simulink model "artedoa_integration_2"  (R2013b)
settings: Solver=ode45  StartTime=0.0  StopTime=1000000  RelTol=1e-3
undefined symbols (not defined in the file or in its folder): calan_lib, comp_addsub
libraries: xbsIndex_r4 x523, casper_library_misc x77, xps_library x1
(part 1 of 2)
settings Model: Creator=root  LastModifiedBy=root

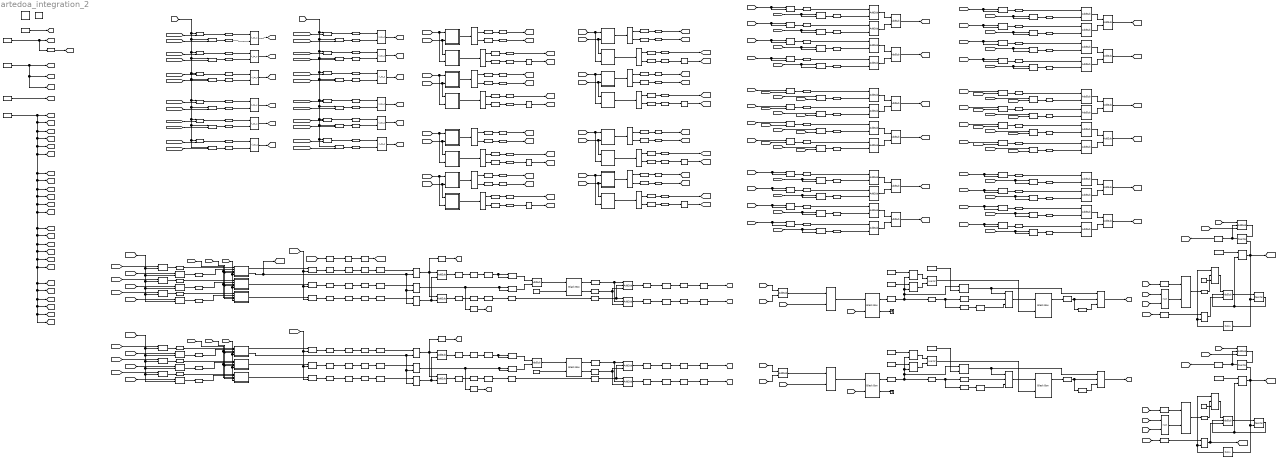
== system artedoa_integration_2 ==
  " System Generator" : xbsIndex_r4/ System Generator  Tag=genX  xilinxfamily=virtex6  part=xc6vsx475t  speed=-1  package=ff1759  synthesis_tool=XST  clock_wrapper=Clock Enables  directory=./doa2dcal/sysgen  proj_type=Project Navigator  Synth_file=XST Defaults  Impl_file=ISE Defaults  testbench=off  simulink_period=1  sysclk_period=7.1429  dcm_input_clock_period=100  incr_netlist=off  trim_vbits=Everywhere in SubSystem  dbl_ovrd=According to Block Masks  core_generation=According to Block Masks  run_coregen=off  deprecated_control=off  eval_field=0  block_type=sysgen
  AddSub : xbsIndex_r4/AddSub  mode=Addition  use_carryin=off  use_carryout=off  en=on  latency=1  precision=User Defined  arith_type="Signed  (2's comp)"  n_bits=26  bin_pt=8  quantization="Round  (unbiased: +/- Inf)"  overflow=Saturate  dbl_ovrd=off  use_behavioral_HDL=off  hw_selection=Fabric  pipelined=off  block_type=addsub
  AddSub1 : xbsIndex_r4/AddSub  mode=Addition  use_carryin=off  use_carryout=off  en=on  latency=1  precision=User Defined  arith_type=Unsigned  n_bits=10  bin_pt=0  quantization="Round  (unbiased: +/- Inf)"  overflow=Saturate  dbl_ovrd=off  use_behavioral_HDL=off  hw_selection=Fabric  pipelined=off  block_type=addsub
  AddSub{2..5,8..11,14..15,18..21,24..25,28..33,36..37} (24 alike) : xbsIndex_r4/AddSub  mode=Addition  use_carryin=off  use_carryout=off  en=off  latency=0  precision=Full  arith_type="Signed  (2's comp)"  n_bits=9  bin_pt=7  quantization="Round  (unbiased: +/- Inf)"  overflow=Saturate  dbl_ovrd=off  use_behavioral_HDL=off  hw_selection=Fabric  pipelined=off  block_type=addsub
  AddSub{6..7,12..13,16..17,22..23,26..27,34..35} (12 alike) : xbsIndex_r4/AddSub  mode=Addition  use_carryin=off  use_carryout=off  en=off  latency=0  precision=Full  arith_type="Signed  (2's comp)"  n_bits=10  bin_pt=7  quantization="Round  (unbiased: +/- Inf)"  overflow=Saturate  dbl_ovrd=off  use_behavioral_HDL=off  hw_selection=Fabric  pipelined=off  block_type=addsub
  AddSub38 : xbsIndex_r4/AddSub  mode=Addition  use_carryin=off  use_carryout=off  en=on  latency=1  precision=User Defined  arith_type="Signed  (2's comp)"  n_bits=26  bin_pt=8  quantization="Round  (unbiased: +/- Inf)"  overflow=Saturate  dbl_ovrd=off  use_behavioral_HDL=off  hw_selection=Fabric  pipelined=off  block_type=addsub
  AddSub39 : xbsIndex_r4/AddSub  mode=Addition  use_carryin=off  use_carryout=off  en=on  latency=1  precision=User Defined  arith_type=Unsigned  n_bits=10  bin_pt=0  quantization="Round  (unbiased: +/- Inf)"  overflow=Saturate  dbl_ovrd=off  use_behavioral_HDL=off  hw_selection=Fabric  pipelined=off  block_type=addsub
  Black Box : xbsIndex_r4/Black Box  init_code=arcsin_config  sim_method=ISE Simulator  verbose=off  block_type=blackbox2
  Black Box1 : xbsIndex_r4/Black Box  init_code=arcsin_config  sim_method=ISE Simulator  verbose=off  block_type=blackbox2
  Constant : xbsIndex_r4/Constant  const=1  gui_display_data_type=Boolean  arith_type=Boolean  n_bits=16  bin_pt=14  preci_type=Single  exp_width=8  frac_width=24  explicit_period=on  period=1  equ=P=C  opselect=C  inp2=PCIN>>17  opr=+  inp1=P  carry=CIN  dbl_ovrd=off  block_type=constant
  Constant1 : xbsIndex_r4/Constant  const=1  gui_display_data_type=Boolean  arith_type=Boolean  n_bits=16  bin_pt=14  preci_type=Single  exp_width=8  frac_width=24  explicit_period=off  period=1  equ=P=C  opselect=C  inp2=PCIN>>17  opr=+  inp1=P  carry=CIN  dbl_ovrd=off  block_type=constant
  Constant10 : xbsIndex_r4/Constant  const=0  gui_display_data_type=Fixed-point  arith_type=Signed (2's comp)  n_bits=16  bin_pt=12  preci_type=Single  exp_width=8  frac_width=24  explicit_period=on  period=1  equ=P=C  opselect=C  inp2=PCIN>>17  opr=+  inp1=P  carry=CIN  dbl_ovrd=off  block_type=constant
  Constant11 : xbsIndex_r4/Constant  const=16  gui_display_data_type=Fixed-point  arith_type=Unsigned  n_bits=10  bin_pt=0  preci_type=Single  exp_width=8  frac_width=24  explicit_period=on  period=1  equ=P=C  opselect=C  inp2=PCIN>>17  opr=+  inp1=P  carry=CIN  dbl_ovrd=off  block_type=constant
  Constant12 : xbsIndex_r4/Constant  const=0  gui_display_data_type=Fixed-point  arith_type=Unsigned  n_bits=1  bin_pt=0  preci_type=Single  exp_width=8  frac_width=24  explicit_period=on  period=1  equ=P=C  opselect=C  inp2=PCIN>>17  opr=+  inp1=P  carry=CIN  dbl_ovrd=off  block_type=constant
  Constant13 : xbsIndex_r4/Constant  const=1  gui_display_data_type=Fixed-point  arith_type=Unsigned  n_bits=7  bin_pt=0  preci_type=Single  exp_width=8  frac_width=24  explicit_period=on  period=1  equ=P=C  opselect=C  inp2=PCIN>>17  opr=+  inp1=P  carry=CIN  dbl_ovrd=off  block_type=constant
  Constant14 : xbsIndex_r4/Constant  const=1  gui_display_data_type=Fixed-point  arith_type=Unsigned  n_bits=9  bin_pt=4  preci_type=Single  exp_width=8  frac_width=24  explicit_period=on  period=1  equ=P=C  opselect=C  inp2=PCIN>>17  opr=+  inp1=P  carry=CIN  dbl_ovrd=off  block_type=constant
  Constant15 : xbsIndex_r4/Constant  const=1  gui_display_data_type=Fixed-point  arith_type=Unsigned  n_bits=18  bin_pt=17  preci_type=Single  exp_width=8  frac_width=24  explicit_period=on  period=1  equ=P=C  opselect=C  inp2=PCIN>>17  opr=+  inp1=P  carry=CIN  dbl_ovrd=off  block_type=constant
  Constant2 : xbsIndex_r4/Constant  const=1  gui_display_data_type=Boolean  arith_type=Boolean  n_bits=16  bin_pt=14  preci_type=Single  exp_width=8  frac_width=24  explicit_period=off  period=1  equ=P=C  opselect=C  inp2=PCIN>>17  opr=+  inp1=P  carry=CIN  dbl_ovrd=off  block_type=constant
  Constant21 : xbsIndex_r4/Constant  const=10000  gui_display_data_type=Fixed-point  arith_type=Unsigned  n_bits=20  bin_pt=0  preci_type=Single  exp_width=8  frac_width=24  explicit_period=on  period=1  equ=P=C  opselect=C  inp2=PCIN>>17  opr=+  inp1=P  carry=CIN  dbl_ovrd=off  block_type=constant
  Constant3 : xbsIndex_r4/Constant  const=1  gui_display_data_type=Fixed-point  arith_type=Signed (2's comp)  n_bits=16  bin_pt=12  preci_type=Single  exp_width=8  frac_width=24  explicit_period=on  period=1  equ=P=C  opselect=C  inp2=PCIN>>17  opr=+  inp1=P  carry=CIN  dbl_ovrd=off  block_type=constant
  Constant4 : xbsIndex_r4/Constant  const=-1  gui_display_data_type=Fixed-point  arith_type=Signed (2's comp)  n_bits=16  bin_pt=12  preci_type=Single  exp_width=8  frac_width=24  explicit_period=on  period=1  equ=P=C  opselect=C  inp2=PCIN>>17  opr=+  inp1=P  carry=CIN  dbl_ovrd=off  block_type=constant
  Constant5 : xbsIndex_r4/Constant  const=0  gui_display_data_type=Fixed-point  arith_type=Signed (2's comp)  n_bits=16  bin_pt=12  preci_type=Single  exp_width=8  frac_width=24  explicit_period=on  period=1  equ=P=C  opselect=C  inp2=PCIN>>17  opr=+  inp1=P  carry=CIN  dbl_ovrd=off  block_type=constant
  Constant6 : xbsIndex_r4/Constant  const=16  gui_display_data_type=Fixed-point  arith_type=Unsigned  n_bits=10  bin_pt=0  preci_type=Single  exp_width=8  frac_width=24  explicit_period=on  period=1  equ=P=C  opselect=C  inp2=PCIN>>17  opr=+  inp1=P  carry=CIN  dbl_ovrd=off  block_type=constant
  Constant7 : xbsIndex_r4/Constant  const=0  gui_display_data_type=Fixed-point  arith_type=Unsigned  n_bits=1  bin_pt=0  preci_type=Single  exp_width=8  frac_width=24  explicit_period=on  period=1  equ=P=C  opselect=C  inp2=PCIN>>17  opr=+  inp1=P  carry=CIN  dbl_ovrd=off  block_type=constant
  Constant8 : xbsIndex_r4/Constant  const=1  gui_display_data_type=Fixed-point  arith_type=Signed (2's comp)  n_bits=16  bin_pt=12  preci_type=Single  exp_width=8  frac_width=24  explicit_period=on  period=1  equ=P=C  opselect=C  inp2=PCIN>>17  opr=+  inp1=P  carry=CIN  dbl_ovrd=off  block_type=constant
  Constant9 : xbsIndex_r4/Constant  const=-1  gui_display_data_type=Fixed-point  arith_type=Signed (2's comp)  n_bits=16  bin_pt=12  preci_type=Single  exp_width=8  frac_width=24  explicit_period=on  period=1  equ=P=C  opselect=C  inp2=PCIN>>17  opr=+  inp1=P  carry=CIN  dbl_ovrd=off  block_type=constant
  Convert{,1..7,9..10,15..19,29..34,41..65,76..77,88,99..116,125..127,130..136,142} (78 alike) : xbsIndex_r4/Convert  gui_display_data_type=Fixed-point  arith_type="Signed  (2's comp)"  n_bits=8  bin_pt=7  float_type=Single  exp_bits=8  fraction_bits=24  quantization="Round  (unbiased: +/- Inf)"  overflow=Saturate  en=off  latency=0  dbl_ovrd=off  pipeline=off  block_type=convert
  Convert{11..14,20..25,66..75,78..87,89..98,117..124} (48 alike) : xbsIndex_r4/Convert  gui_display_data_type=Fixed-point  arith_type="Signed  (2's comp)"  n_bits=15  bin_pt=14  float_type=Single  exp_bits=8  fraction_bits=24  quantization="Round  (unbiased: +/- Inf)"  overflow=Saturate  en=off  latency=0  dbl_ovrd=off  pipeline=off  block_type=convert
  Convert{26,38,128,140} (4 alike) : xbsIndex_r4/Convert  gui_display_data_type=Fixed-point  arith_type="Signed  (2's comp)"  n_bits=15  bin_pt=6  float_type=Single  exp_bits=8  fraction_bits=24  quantization="Round  (unbiased: +/- Inf)"  overflow=Saturate  en=off  latency=0  dbl_ovrd=off  pipeline=off  block_type=convert
  Convert{27,39,129,141} (4 alike) : xbsIndex_r4/Convert  gui_display_data_type=Fixed-point  arith_type="Signed  (2's comp)"  n_bits=9  bin_pt=8  float_type=Single  exp_bits=8  fraction_bits=24  quantization="Round  (unbiased: +/- Inf)"  overflow=Saturate  en=off  latency=0  dbl_ovrd=off  pipeline=off  block_type=convert
  Convert{35..37,137..139} (6 alike) : xbsIndex_r4/Convert  gui_display_data_type=Fixed-point  arith_type="Signed  (2's comp)"  n_bits=28  bin_pt=7  float_type=Single  exp_bits=8  fraction_bits=24  quantization="Round  (unbiased: +/- Inf)"  overflow=Saturate  en=off  latency=0  dbl_ovrd=off  pipeline=off  block_type=convert
  Convert143 : xbsIndex_r4/Convert  gui_display_data_type=Boolean  arith_type=Boolean  n_bits=8  bin_pt=0  float_type=Single  exp_bits=8  fraction_bits=24  quantization="Round  (unbiased: +/- Inf)"  overflow=Saturate  en=off  latency=0  dbl_ovrd=off  pipeline=off  block_type=convert
  Convert144 : xbsIndex_r4/Convert  gui_display_data_type=Fixed-point  arith_type="Signed  (2's comp)"  n_bits=13  bin_pt=12  float_type=Single  exp_bits=8  fraction_bits=24  quantization="Round  (unbiased: +/- Inf)"  overflow=Saturate  en=off  latency=0  dbl_ovrd=off  pipeline=off  block_type=convert
  Convert145 : xbsIndex_r4/Convert  gui_display_data_type=Fixed-point  arith_type=Unsigned  n_bits=1  bin_pt=0  float_type=Single  exp_bits=8  fraction_bits=24  quantization="Round  (unbiased: +/- Inf)"  overflow=Saturate  en=off  latency=0  dbl_ovrd=off  pipeline=off  block_type=convert
  Convert28 : xbsIndex_r4/Convert  gui_display_data_type=Fixed-point  arith_type="Signed  (2's comp)"  n_bits=13  bin_pt=12  float_type=Single  exp_bits=8  fraction_bits=24  quantization="Round  (unbiased: +/- Inf)"  overflow=Saturate  en=off  latency=0  dbl_ovrd=off  pipeline=off  block_type=convert
  Convert40 : xbsIndex_r4/Convert  gui_display_data_type=Fixed-point  arith_type=Unsigned  n_bits=1  bin_pt=0  float_type=Single  exp_bits=8  fraction_bits=24  quantization="Round  (unbiased: +/- Inf)"  overflow=Saturate  en=off  latency=0  dbl_ovrd=off  pipeline=off  block_type=convert
  Convert8 : xbsIndex_r4/Convert  gui_display_data_type=Boolean  arith_type=Boolean  n_bits=8  bin_pt=0  float_type=Single  exp_bits=8  fraction_bits=24  quantization="Round  (unbiased: +/- Inf)"  overflow=Saturate  en=off  latency=0  dbl_ovrd=off  pipeline=off  block_type=convert
  Delay{,3,10..11,17..18} (6 alike) : xbsIndex_r4/Delay  rst=off  infoeditControl=Selection of Reset will increase slice count due to use of real FFs and instead of SRLs  en=off  latency=3  dbl_ovrd=off  reg_retiming=off  block_type=delay
  Delay{1,4,9,19} (4 alike) : xbsIndex_r4/Delay  rst=off  infoeditControl=Selection of Reset will increase slice count due to use of real FFs and instead of SRLs  en=off  latency=1  dbl_ovrd=off  reg_retiming=off  block_type=delay
  Delay{2,5..8,12..13} (7 alike) : xbsIndex_r4/Delay  rst=off  infoeditControl=Selection of Reset will increase slice count due to use of real FFs and instead of SRLs  en=off  latency=4  dbl_ovrd=off  reg_retiming=off  block_type=delay
  Logical : xbsIndex_r4/Logical  logical_function=OR  inputs=2  en=off  latency=0  precision=Full  arith_type=Unsigned  n_bits=16  bin_pt=0  align_bp=on  dbl_ovrd=off  block_type=logical
  Logical1 : xbsIndex_r4/Logical  logical_function=AND  inputs=2  en=off  latency=0  precision=Full  arith_type=Unsigned  n_bits=16  bin_pt=0  align_bp=on  dbl_ovrd=off  block_type=logical
  Logical2 : xbsIndex_r4/Logical  logical_function=AND  inputs=2  en=off  latency=0  precision=Full  arith_type=Unsigned  n_bits=16  bin_pt=0  align_bp=on  dbl_ovrd=off  block_type=logical
  Logical3 : xbsIndex_r4/Logical  logical_function=OR  inputs=2  en=off  latency=0  precision=Full  arith_type=Unsigned  n_bits=16  bin_pt=0  align_bp=on  dbl_ovrd=off  block_type=logical
  Mult{,0..11,14..84,87..94} (92 alike) : xbsIndex_r4/Mult  precision=Full  arith_type="Signed  (2's comp)"  n_bits=16  bin_pt=14  quantization=Truncate  overflow=Wrap  en=off  latency=3  dbl_ovrd=off  use_behavioral_HDL=off  opt=Speed  use_embedded=on  optimum_pipeline=off  pipeline=on  use_rpm=on  placement_style=Triangular  block_type=mult
  Mult{12..13,85..86} (4 alike) : xbsIndex_r4/Mult  precision=User Defined  arith_type=Unsigned  n_bits=16  bin_pt=0  quantization="Round  (unbiased: +/- Inf)"  overflow=Saturate  en=off  latency=3  dbl_ovrd=off  use_behavioral_HDL=off  opt=Speed  use_embedded=on  optimum_pipeline=off  pipeline=on  use_rpm=on  placement_style=Triangular  block_type=mult
  Mux{,1..5} (6 alike) : xbsIndex_r4/Mux  inputs=2  en=off  latency=0  precision=Full  arith_type=Unsigned  n_bits=16  bin_pt=14  quantization=Truncate  overflow=Wrap  dbl_ovrd=off  block_type=mux
  Mx{1..3,11..12,22} (6 alike) : xbsIndex_r4/Register  init=0  rst=off  en=on  dbl_ovrd=off  block_type=register
  Negate{,1,4..9} (8 alike) : xbsIndex_r4/Negate  precision=User Defined  arith_type="Signed  (2's comp)"  n_bits=8  bin_pt=7  quantization="Round  (unbiased: +/- Inf)"  overflow=Saturate  en=off  latency=0  dbl_ovrd=off  block_type=negate
  Negate10 : xbsIndex_r4/Negate  precision=User Defined  arith_type="Signed  (2's comp)"  n_bits=13  bin_pt=12  quantization="Round  (unbiased: +/- Inf)"  overflow=Saturate  en=off  latency=0  dbl_ovrd=off  block_type=negate
  Negate11 : xbsIndex_r4/Negate  precision=User Defined  arith_type="Signed  (2's comp)"  n_bits=16  bin_pt=8  quantization="Round  (unbiased: +/- Inf)"  overflow=Saturate  en=off  latency=0  dbl_ovrd=off  block_type=negate
  Negate2 : xbsIndex_r4/Negate  precision=User Defined  arith_type="Signed  (2's comp)"  n_bits=13  bin_pt=12  quantization="Round  (unbiased: +/- Inf)"  overflow=Saturate  en=off  latency=0  dbl_ovrd=off  block_type=negate
  Negate3 : xbsIndex_r4/Negate  precision=User Defined  arith_type="Signed  (2's comp)"  n_bits=16  bin_pt=8  quantization="Round  (unbiased: +/- Inf)"  overflow=Saturate  en=off  latency=0  dbl_ovrd=off  block_type=negate
  Register{,1..3} (4 alike) : xbsIndex_r4/Register  init=0  rst=on  en=off  dbl_ovrd=off  block_type=register
  Reinterpret : xbsIndex_r4/Reinterpret  force_arith_type=off  arith_type=Unsigned  force_bin_pt=on  bin_pt=6  block_type=reinterpret
  Reinterpret{1,3,52,59} (4 alike) : xbsIndex_r4/Reinterpret  force_arith_type=off  arith_type=Unsigned  force_bin_pt=on  bin_pt=8  block_type=reinterpret
  Reinterpret{6,8,10,53,62,64} (6 alike) : xbsIndex_r4/Reinterpret  force_arith_type=on  arith_type="Signed  (2's comp)"  force_bin_pt=on  bin_pt=0  block_type=reinterpret
  Reinterpret{11..14,22..50,66} (34 alike) : xbsIndex_r4/Reinterpret  force_arith_type=on  arith_type="Signed  (2's comp)"  force_bin_pt=on  bin_pt=8  block_type=reinterpret
  Reinterpret{15,20,54,57} (4 alike) : xbsIndex_r4/Reinterpret  force_arith_type=off  arith_type=Unsigned  force_bin_pt=on  bin_pt=14  block_type=reinterpret
  Reinterpret{2,4,16,21,55..56,58,60} (8 alike) : xbsIndex_r4/Reinterpret  force_arith_type=off  arith_type=Unsigned  force_bin_pt=on  bin_pt=0  block_type=reinterpret
  Reinterpret17 : xbsIndex_r4/Reinterpret  force_arith_type=on  arith_type="Signed  (2's comp)"  force_bin_pt=on  bin_pt=12  block_type=reinterpret
  Reinterpret{18..19,68..69} (4 alike) : xbsIndex_r4/Reinterpret  force_arith_type=on  arith_type=Unsigned  force_bin_pt=on  bin_pt=0  block_type=reinterpret
  Reinterpret{5,7,9,61,63,65} (6 alike) : xbsIndex_r4/Reinterpret  force_arith_type=on  arith_type="Signed  (2's comp)"  force_bin_pt=on  bin_pt=27  block_type=reinterpret
  Reinterpret51 : xbsIndex_r4/Reinterpret  force_arith_type=off  arith_type=Unsigned  force_bin_pt=on  bin_pt=6  block_type=reinterpret
  Reinterpret67 : xbsIndex_r4/Reinterpret  force_arith_type=on  arith_type="Signed  (2's comp)"  force_bin_pt=on  bin_pt=12  block_type=reinterpret
  Relational : xbsIndex_r4/Relational  mode=a>=b  en=off  latency=0  dbl_ovrd=off  block_type=relational
  Relational{1..2,6..7} (4 alike) : xbsIndex_r4/Relational  mode=a<=b  en=off  latency=0  dbl_ovrd=off  block_type=relational
  Relational3 : xbsIndex_r4/Relational  mode=a>b  en=off  latency=0  dbl_ovrd=off  block_type=relational
  Relational4 : xbsIndex_r4/Relational  mode=a=b  en=off  latency=0  dbl_ovrd=off  block_type=relational
  Relational5 : xbsIndex_r4/Relational  mode=a>=b  en=off  latency=0  dbl_ovrd=off  block_type=relational
  Relational8 : xbsIndex_r4/Relational  mode=a>b  en=off  latency=0  dbl_ovrd=off  block_type=relational
  Relational9 : xbsIndex_r4/Relational  mode=a=b  en=off  latency=0  dbl_ovrd=off  block_type=relational
  Shift : xbsIndex_r4/Shift  shift_dir=Right  shift_bits=4  en=off  latency=0  precision=Full  arith_type="Signed  (2's comp)"  n_bits=16  bin_pt=14  quantization=Truncate  overflow=Wrap  dbl_ovrd=off  block_type=shift
  Shift1 : xbsIndex_r4/Shift  shift_dir=Right  shift_bits=4  en=off  latency=0  precision=Full  arith_type="Signed  (2's comp)"  n_bits=16  bin_pt=14  quantization=Truncate  overflow=Wrap  dbl_ovrd=off  block_type=shift
  Subsystem1 : Subsystem
  Subsystem16 : Subsystem
  Subsystem17 : Subsystem
  Subsystem2 : Subsystem
  Subsystem3 : Subsystem
  Subsystem4 : Subsystem
  Terminator : Terminator
  Terminator1 : Terminator
  XSG_core_config : xps_library/XSG_core_config  Tag=xps:xsg  hw_sys=ROACH2:sx475t  clk_src=adc0_clk  ROACH_clk_src=sys_clk  ROACH2_clk_src=adc0_clk  MKDIG_clk_src=sys_clk  clk_rate=140  sample_period=1  synthesis_tool=XST
  a_c1 : xbsIndex_r4/AddSub  mode=Subtraction  use_carryin=off  use_carryout=off  en=off  latency=0  precision=Full  arith_type="Signed  (2's comp)"  n_bits=64  bin_pt=26  quantization="Round  (unbiased: +/- Inf)"  overflow=Wrap  dbl_ovrd=off  use_behavioral_HDL=off  hw_selection=Fabric  pipelined=off  block_type=addsub
  a_c2 : xbsIndex_r4/AddSub  mode=Subtraction  use_carryin=off  use_carryout=off  en=off  latency=0  precision=Full  arith_type="Signed  (2's comp)"  n_bits=64  bin_pt=26  quantization="Round  (unbiased: +/- Inf)"  overflow=Wrap  dbl_ovrd=off  use_behavioral_HDL=off  hw_selection=Fabric  pipelined=off  block_type=addsub
  arctan : xbsIndex_r4/Black Box  init_code=arctan2_config  sim_method=ISE Simulator  verbose=off  block_type=blackbox2
  arctan1 : xbsIndex_r4/Black Box  init_code=arctan2_config  sim_method=ISE Simulator  verbose=off  block_type=blackbox2
  bus_create : Subsystem  AncestorBlock=casper_library_flow_control/bus_create  mask(bus_create){inputNum=2}
      mask prompts: inputNum "Number of inputs:"
      mask init:
      | bus_create_init(gcb,...
      |     'inputNum', inputNum);
  bus_create1 : Subsystem  AncestorBlock=casper_library_flow_control/bus_create  mask(bus_create){inputNum=2}
      mask prompts: inputNum "Number of inputs:"
      mask init:
      | bus_create_init(gcb,...
      |     'inputNum', inputNum);
  c_to_ri{,1..15} (16 alike) : casper_library_misc/c_to_ri  n_bits=9  bin_pt=7
      settings: AttributesFormatString=9_7 r/i
  comp_addsub : Subsystem  AncestorBlock=calan_lib/comp_addsub  mask(comp_addsub){addsub=Addition, n_bits_in=8, bin_pt_in=7, add_latency=2, n_bits_out=9, bin_pt_out=7, quantization=Round  (unbiased: +/- Inf), overflow=Saturate}
      mask prompts: addsub "Addition/Subtraction"; n_bits_in "Bit Width"; bin_pt_in "Binary Point"; add_latency "Adder Latency"; n_bits_out "Bit Width"; bin_pt_out "BInary Point"
      mask help: Add or substract two complex numbers of the same length.
      mask init:
      | comp_addsub_init(gcb, ...
      |     'addsub', addsub, ...
      |     'n_bits_in', n_bits_in, ...
      |     'bin_pt_in', bin_pt_in, ...
      |     'n_bits_out', n_bits_out, ...
      |     'bin_pt_out', bin_pt_out, ...
      |     'quantization', quantization, ...
      |     'overflow', overflow, ...
      |     'add_latency', add_latency);
      settings: AttributesFormatString=|
      | 8_7 * 8_7 ==> 9_7
      | Round  (unbiased: +/- Inf), Saturate
      mask TypeOptions addsub: Addition | Subtraction
      mask TypeOptions quantization: Truncate | Round  (unbiased: +/- Inf)
      mask TypeOptions overflow: Wrap | Saturate | Flag as error
      mask Display:
      | port_label('input', 1, 'a');
      | port_label('input', 2, 'b');
      | if strcmp(addsub, 'Addition')
      |     port_label('output', 1, 'a+b');
      | elseif strcmp(addsub, 'Subtraction')
      |     port_label('output', 1, 'a-b');
      | end
      | disp(['Z^-', num2str(add_latency)]);
  comp_addsub1 : Subsystem  AncestorBlock=calan_lib/comp_addsub  mask(comp_addsub){addsub=Subtraction, n_bits_in=8, bin_pt_in=7, add_latency=2, n_bits_out=9, bin_pt_out=7, quantization=Round  (unbiased: +/- Inf), overflow=Saturate}
      mask prompts: addsub "Addition/Subtraction"; n_bits_in "Bit Width"; bin_pt_in "Binary Point"; add_latency "Adder Latency"; n_bits_out "Bit Width"; bin_pt_out "BInary Point"
      mask help: Add or substract two complex numbers of the same length.
      mask init: same as artedoa_integration_2/comp_addsub
      settings: AttributesFormatString=|
      | 8_7 * 8_7 ==> 9_7
      | Round  (unbiased: +/- Inf), Saturate
      mask TypeOptions addsub: Addition | Subtraction
      mask TypeOptions quantization: Truncate | Round  (unbiased: +/- Inf)
      mask TypeOptions overflow: Wrap | Saturate | Flag as error
      mask Display:
      | port_label('input', 1, 'a');
      | port_label('input', 2, 'b');
      | if strcmp(addsub, 'Addition')
      |     port_label('output', 1, 'a+b');
      | elseif strcmp(addsub, 'Subtraction')
      |     port_label('output', 1, 'a-b');
      | end
      | disp(['Z^-', num2str(add_latency)]);
  comp_addsub10 : Subsystem  AncestorBlock=calan_lib/comp_addsub  mask(comp_addsub){addsub=Addition, n_bits_in=8, bin_pt_in=7, add_latency=2, n_bits_out=9, bin_pt_out=7, quantization=Round  (unbiased: +/- Inf), overflow=Saturate}
      mask prompts: addsub "Addition/Subtraction"; n_bits_in "Bit Width"; bin_pt_in "Binary Point"; add_latency "Adder Latency"; n_bits_out "Bit Width"; bin_pt_out "BInary Point"
      mask help: Add or substract two complex numbers of the same length.
      mask init: same as artedoa_integration_2/comp_addsub
      settings: AttributesFormatString=|
      | 8_7 * 8_7 ==> 9_7
      | Round  (unbiased: +/- Inf), Saturate
      mask TypeOptions addsub: Addition | Subtraction
      mask TypeOptions quantization: Truncate | Round  (unbiased: +/- Inf)
      mask TypeOptions overflow: Wrap | Saturate | Flag as error
      mask Display:
      | port_label('input', 1, 'a');
      | port_label('input', 2, 'b');
      | if strcmp(addsub, 'Addition')
      |     port_label('output', 1, 'a+b');
      | elseif strcmp(addsub, 'Subtraction')
      |     port_label('output', 1, 'a-b');
      | end
      | disp(['Z^-', num2str(add_latency)]);
  comp_addsub11 : Subsystem  AncestorBlock=calan_lib/comp_addsub  mask(comp_addsub){addsub=Subtraction, n_bits_in=8, bin_pt_in=7, add_latency=2, n_bits_out=9, bin_pt_out=7, quantization=Round  (unbiased: +/- Inf), overflow=Saturate}
      mask prompts: addsub "Addition/Subtraction"; n_bits_in "Bit Width"; bin_pt_in "Binary Point"; add_latency "Adder Latency"; n_bits_out "Bit Width"; bin_pt_out "BInary Point"
      mask help: Add or substract two complex numbers of the same length.
      mask init: same as artedoa_integration_2/comp_addsub
      settings: AttributesFormatString=|
      | 8_7 * 8_7 ==> 9_7
      | Round  (unbiased: +/- Inf), Saturate
      mask TypeOptions addsub: Addition | Subtraction
      mask TypeOptions quantization: Truncate | Round  (unbiased: +/- Inf)
      mask TypeOptions overflow: Wrap | Saturate | Flag as error
      mask Display:
      | port_label('input', 1, 'a');
      | port_label('input', 2, 'b');
      | if strcmp(addsub, 'Addition')
      |     port_label('output', 1, 'a+b');
      | elseif strcmp(addsub, 'Subtraction')
      |     port_label('output', 1, 'a-b');
      | end
      | disp(['Z^-', num2str(add_latency)]);
  comp_addsub12 : Subsystem  AncestorBlock=calan_lib/comp_addsub  mask(comp_addsub){addsub=Addition, n_bits_in=8, bin_pt_in=7, add_latency=2, n_bits_out=9, bin_pt_out=7, quantization=Round  (unbiased: +/- Inf), overflow=Saturate}
      mask prompts: addsub "Addition/Subtraction"; n_bits_in "Bit Width"; bin_pt_in "Binary Point"; add_latency "Adder Latency"; n_bits_out "Bit Width"; bin_pt_out "BInary Point"
      mask help: Add or substract two complex numbers of the same length.
      mask init: same as artedoa_integration_2/comp_addsub
      settings: AttributesFormatString=|
      | 8_7 * 8_7 ==> 9_7
      | Round  (unbiased: +/- Inf), Saturate
      mask TypeOptions addsub: Addition | Subtraction
      mask TypeOptions quantization: Truncate | Round  (unbiased: +/- Inf)
      mask TypeOptions overflow: Wrap | Saturate | Flag as error
      mask Display:
      | port_label('input', 1, 'a');
      | port_label('input', 2, 'b');
      | if strcmp(addsub, 'Addition')
      |     port_label('output', 1, 'a+b');
      | elseif strcmp(addsub, 'Subtraction')
      |     port_label('output', 1, 'a-b');
      | end
      | disp(['Z^-', num2str(add_latency)]);
  comp_addsub13 : Subsystem  AncestorBlock=calan_lib/comp_addsub  mask(comp_addsub){addsub=Subtraction, n_bits_in=8, bin_pt_in=7, add_latency=2, n_bits_out=9, bin_pt_out=7, quantization=Round  (unbiased: +/- Inf), overflow=Saturate}
      mask prompts: addsub "Addition/Subtraction"; n_bits_in "Bit Width"; bin_pt_in "Binary Point"; add_latency "Adder Latency"; n_bits_out "Bit Width"; bin_pt_out "BInary Point"
      mask help: Add or substract two complex numbers of the same length.
      mask init: same as artedoa_integration_2/comp_addsub
      settings: AttributesFormatString=|
      | 8_7 * 8_7 ==> 9_7
      | Round  (unbiased: +/- Inf), Saturate
      mask TypeOptions addsub: Addition | Subtraction
      mask TypeOptions quantization: Truncate | Round  (unbiased: +/- Inf)
      mask TypeOptions overflow: Wrap | Saturate | Flag as error
      mask Display:
      | port_label('input', 1, 'a');
      | port_label('input', 2, 'b');
      | if strcmp(addsub, 'Addition')
      |     port_label('output', 1, 'a+b');
      | elseif strcmp(addsub, 'Subtraction')
      |     port_label('output', 1, 'a-b');
      | end
      | disp(['Z^-', num2str(add_latency)]);
  comp_addsub14 : Subsystem  AncestorBlock=calan_lib/comp_addsub  mask(comp_addsub){addsub=Addition, n_bits_in=8, bin_pt_in=7, add_latency=2, n_bits_out=9, bin_pt_out=7, quantization=Round  (unbiased: +/- Inf), overflow=Saturate}
      mask prompts: addsub "Addition/Subtraction"; n_bits_in "Bit Width"; bin_pt_in "Binary Point"; add_latency "Adder Latency"; n_bits_out "Bit Width"; bin_pt_out "BInary Point"
      mask help: Add or substract two complex numbers of the same length.
      mask init: same as artedoa_integration_2/comp_addsub
      settings: AttributesFormatString=|
      | 8_7 * 8_7 ==> 9_7
      | Round  (unbiased: +/- Inf), Saturate
      mask TypeOptions addsub: Addition | Subtraction
      mask TypeOptions quantization: Truncate | Round  (unbiased: +/- Inf)
      mask TypeOptions overflow: Wrap | Saturate | Flag as error
      mask Display:
      | port_label('input', 1, 'a');
      | port_label('input', 2, 'b');
      | if strcmp(addsub, 'Addition')
      |     port_label('output', 1, 'a+b');
      | elseif strcmp(addsub, 'Subtraction')
      |     port_label('output', 1, 'a-b');
      | end
      | disp(['Z^-', num2str(add_latency)]);
  comp_addsub15 : Subsystem  AncestorBlock=calan_lib/comp_addsub  mask(comp_addsub){addsub=Subtraction, n_bits_in=8, bin_pt_in=7, add_latency=2, n_bits_out=9, bin_pt_out=7, quantization=Round  (unbiased: +/- Inf), overflow=Saturate}
      mask prompts: addsub "Addition/Subtraction"; n_bits_in "Bit Width"; bin_pt_in "Binary Point"; add_latency "Adder Latency"; n_bits_out "Bit Width"; bin_pt_out "BInary Point"
      mask help: Add or substract two complex numbers of the same length.
      mask init: same as artedoa_integration_2/comp_addsub
      settings: AttributesFormatString=|
      | 8_7 * 8_7 ==> 9_7
      | Round  (unbiased: +/- Inf), Saturate
      mask TypeOptions addsub: Addition | Subtraction
      mask TypeOptions quantization: Truncate | Round  (unbiased: +/- Inf)
      mask TypeOptions overflow: Wrap | Saturate | Flag as error
      mask Display:
      | port_label('input', 1, 'a');
      | port_label('input', 2, 'b');
      | if strcmp(addsub, 'Addition')
      |     port_label('output', 1, 'a+b');
      | elseif strcmp(addsub, 'Subtraction')
      |     port_label('output', 1, 'a-b');
      | end
      | disp(['Z^-', num2str(add_latency)]);
  comp_addsub2 : Subsystem  AncestorBlock=calan_lib/comp_addsub  mask(comp_addsub){addsub=Addition, n_bits_in=8, bin_pt_in=7, add_latency=2, n_bits_out=9, bin_pt_out=7, quantization=Round  (unbiased: +/- Inf), overflow=Saturate}
      mask prompts: addsub "Addition/Subtraction"; n_bits_in "Bit Width"; bin_pt_in "Binary Point"; add_latency "Adder Latency"; n_bits_out "Bit Width"; bin_pt_out "BInary Point"
      mask help: Add or substract two complex numbers of the same length.
      mask init: same as artedoa_integration_2/comp_addsub
      settings: AttributesFormatString=|
      | 8_7 * 8_7 ==> 9_7
      | Round  (unbiased: +/- Inf), Saturate
      mask TypeOptions addsub: Addition | Subtraction
      mask TypeOptions quantization: Truncate | Round  (unbiased: +/- Inf)
      mask TypeOptions overflow: Wrap | Saturate | Flag as error
      mask Display:
      | port_label('input', 1, 'a');
      | port_label('input', 2, 'b');
      | if strcmp(addsub, 'Addition')
      |     port_label('output', 1, 'a+b');
      | elseif strcmp(addsub, 'Subtraction')
      |     port_label('output', 1, 'a-b');
      | end
      | disp(['Z^-', num2str(add_latency)]);
  comp_addsub3 : Subsystem  AncestorBlock=calan_lib/comp_addsub  mask(comp_addsub){addsub=Subtraction, n_bits_in=8, bin_pt_in=7, add_latency=2, n_bits_out=9, bin_pt_out=7, quantization=Round  (unbiased: +/- Inf), overflow=Saturate}
      mask prompts: addsub "Addition/Subtraction"; n_bits_in "Bit Width"; bin_pt_in "Binary Point"; add_latency "Adder Latency"; n_bits_out "Bit Width"; bin_pt_out "BInary Point"
      mask help: Add or substract two complex numbers of the same length.
      mask init: same as artedoa_integration_2/comp_addsub
      settings: AttributesFormatString=|
      | 8_7 * 8_7 ==> 9_7
      | Round  (unbiased: +/- Inf), Saturate
      mask TypeOptions addsub: Addition | Subtraction
      mask TypeOptions quantization: Truncate | Round  (unbiased: +/- Inf)
      mask TypeOptions overflow: Wrap | Saturate | Flag as error
      mask Display:
      | port_label('input', 1, 'a');
      | port_label('input', 2, 'b');
      | if strcmp(addsub, 'Addition')
      |     port_label('output', 1, 'a+b');
      | elseif strcmp(addsub, 'Subtraction')
      |     port_label('output', 1, 'a-b');
      | end
      | disp(['Z^-', num2str(add_latency)]);
  comp_addsub4 : Subsystem  AncestorBlock=calan_lib/comp_addsub  mask(comp_addsub){addsub=Addition, n_bits_in=8, bin_pt_in=7, add_latency=2, n_bits_out=9, bin_pt_out=7, quantization=Round  (unbiased: +/- Inf), overflow=Saturate}
      mask prompts: addsub "Addition/Subtraction"; n_bits_in "Bit Width"; bin_pt_in "Binary Point"; add_latency "Adder Latency"; n_bits_out "Bit Width"; bin_pt_out "BInary Point"
      mask help: Add or substract two complex numbers of the same length.
      mask init: same as artedoa_integration_2/comp_addsub
      settings: AttributesFormatString=|
      | 8_7 * 8_7 ==> 9_7
      | Round  (unbiased: +/- Inf), Saturate
      mask TypeOptions addsub: Addition | Subtraction
      mask TypeOptions quantization: Truncate | Round  (unbiased: +/- Inf)
      mask TypeOptions overflow: Wrap | Saturate | Flag as error
      mask Display:
      | port_label('input', 1, 'a');
      | port_label('input', 2, 'b');
      | if strcmp(addsub, 'Addition')
      |     port_label('output', 1, 'a+b');
      | elseif strcmp(addsub, 'Subtraction')
      |     port_label('output', 1, 'a-b');
      | end
      | disp(['Z^-', num2str(add_latency)]);
  comp_addsub5 : Subsystem  AncestorBlock=calan_lib/comp_addsub  mask(comp_addsub){addsub=Subtraction, n_bits_in=8, bin_pt_in=7, add_latency=2, n_bits_out=9, bin_pt_out=7, quantization=Round  (unbiased: +/- Inf), overflow=Saturate}
      mask prompts: addsub "Addition/Subtraction"; n_bits_in "Bit Width"; bin_pt_in "Binary Point"; add_latency "Adder Latency"; n_bits_out "Bit Width"; bin_pt_out "BInary Point"
      mask help: Add or substract two complex numbers of the same length.
      mask init: same as artedoa_integration_2/comp_addsub
      settings: AttributesFormatString=|
      | 8_7 * 8_7 ==> 9_7
      | Round  (unbiased: +/- Inf), Saturate
      mask TypeOptions addsub: Addition | Subtraction
      mask TypeOptions quantization: Truncate | Round  (unbiased: +/- Inf)
      mask TypeOptions overflow: Wrap | Saturate | Flag as error
      mask Display:
      | port_label('input', 1, 'a');
      | port_label('input', 2, 'b');
      | if strcmp(addsub, 'Addition')
      |     port_label('output', 1, 'a+b');
      | elseif strcmp(addsub, 'Subtraction')
      |     port_label('output', 1, 'a-b');
      | end
      | disp(['Z^-', num2str(add_latency)]);
  comp_addsub6 : Subsystem  AncestorBlock=calan_lib/comp_addsub  mask(comp_addsub){addsub=Addition, n_bits_in=8, bin_pt_in=7, add_latency=2, n_bits_out=9, bin_pt_out=7, quantization=Round  (unbiased: +/- Inf), overflow=Saturate}
      mask prompts: addsub "Addition/Subtraction"; n_bits_in "Bit Width"; bin_pt_in "Binary Point"; add_latency "Adder Latency"; n_bits_out "Bit Width"; bin_pt_out "BInary Point"
      mask help: Add or substract two complex numbers of the same length.
      mask init: same as artedoa_integration_2/comp_addsub
      settings: AttributesFormatString=|
      | 8_7 * 8_7 ==> 9_7
      | Round  (unbiased: +/- Inf), Saturate
      mask TypeOptions addsub: Addition | Subtraction
      mask TypeOptions quantization: Truncate | Round  (unbiased: +/- Inf)
      mask TypeOptions overflow: Wrap | Saturate | Flag as error
      mask Display:
      | port_label('input', 1, 'a');
      | port_label('input', 2, 'b');
      | if strcmp(addsub, 'Addition')
      |     port_label('output', 1, 'a+b');
      | elseif strcmp(addsub, 'Subtraction')
      |     port_label('output', 1, 'a-b');
      | end
      | disp(['Z^-', num2str(add_latency)]);
  comp_addsub7 : Subsystem  AncestorBlock=calan_lib/comp_addsub  mask(comp_addsub){addsub=Subtraction, n_bits_in=8, bin_pt_in=7, add_latency=2, n_bits_out=9, bin_pt_out=7, quantization=Round  (unbiased: +/- Inf), overflow=Saturate}
      mask prompts: addsub "Addition/Subtraction"; n_bits_in "Bit Width"; bin_pt_in "Binary Point"; add_latency "Adder Latency"; n_bits_out "Bit Width"; bin_pt_out "BInary Point"
      mask help: Add or substract two complex numbers of the same length.
      mask init: same as artedoa_integration_2/comp_addsub
      settings: AttributesFormatString=|
      | 8_7 * 8_7 ==> 9_7
      | Round  (unbiased: +/- Inf), Saturate
      mask TypeOptions addsub: Addition | Subtraction
      mask TypeOptions quantization: Truncate | Round  (unbiased: +/- Inf)
      mask TypeOptions overflow: Wrap | Saturate | Flag as error
      mask Display:
      | port_label('input', 1, 'a');
      | port_label('input', 2, 'b');
      | if strcmp(addsub, 'Addition')
      |     port_label('output', 1, 'a+b');
      | elseif strcmp(addsub, 'Subtraction')
      |     port_label('output', 1, 'a-b');
      | end
      | disp(['Z^-', num2str(add_latency)]);
  comp_addsub8 : Subsystem  AncestorBlock=calan_lib/comp_addsub  mask(comp_addsub){addsub=Addition, n_bits_in=8, bin_pt_in=7, add_latency=2, n_bits_out=9, bin_pt_out=7, quantization=Round  (unbiased: +/- Inf), overflow=Saturate}
      mask prompts: addsub "Addition/Subtraction"; n_bits_in "Bit Width"; bin_pt_in "Binary Point"; add_latency "Adder Latency"; n_bits_out "Bit Width"; bin_pt_out "BInary Point"
      mask help: Add or substract two complex numbers of the same length.
      mask init: same as artedoa_integration_2/comp_addsub
      settings: AttributesFormatString=|
      | 8_7 * 8_7 ==> 9_7
      | Round  (unbiased: +/- Inf), Saturate
      mask TypeOptions addsub: Addition | Subtraction
      mask TypeOptions quantization: Truncate | Round  (unbiased: +/- Inf)
      mask TypeOptions overflow: Wrap | Saturate | Flag as error
      mask Display:
      | port_label('input', 1, 'a');
      | port_label('input', 2, 'b');
      | if strcmp(addsub, 'Addition')
      |     port_label('output', 1, 'a+b');
      | elseif strcmp(addsub, 'Subtraction')
      |     port_label('output', 1, 'a-b');
      | end
      | disp(['Z^-', num2str(add_latency)]);
  comp_addsub9 : Subsystem  AncestorBlock=calan_lib/comp_addsub  mask(comp_addsub){addsub=Subtraction, n_bits_in=8, bin_pt_in=7, add_latency=2, n_bits_out=9, bin_pt_out=7, quantization=Round  (unbiased: +/- Inf), overflow=Saturate}
      mask prompts: addsub "Addition/Subtraction"; n_bits_in "Bit Width"; bin_pt_in "Binary Point"; add_latency "Adder Latency"; n_bits_out "Bit Width"; bin_pt_out "BInary Point"
      mask help: Add or substract two complex numbers of the same length.
      mask init: same as artedoa_integration_2/comp_addsub
      settings: AttributesFormatString=|
      | 8_7 * 8_7 ==> 9_7
      | Round  (unbiased: +/- Inf), Saturate
      mask TypeOptions addsub: Addition | Subtraction
      mask TypeOptions quantization: Truncate | Round  (unbiased: +/- Inf)
      mask TypeOptions overflow: Wrap | Saturate | Flag as error
      mask Display:
      | port_label('input', 1, 'a');
      | port_label('input', 2, 'b');
      | if strcmp(addsub, 'Addition')
      |     port_label('output', 1, 'a+b');
      | elseif strcmp(addsub, 'Subtraction')
      |     port_label('output', 1, 'a-b');
      | end
      | disp(['Z^-', num2str(add_latency)]);
  edge_detect1 : casper_library_misc/edge_detect  edge=Rising  polarity=Active High  x_in=[0 0.08 0.08 0.16 0.16 0.24 0.24 0.32 0.32 0.4]  y_in="[-1 -1  1  1  1  1  1  1  1  1]"  x_out=[0.6 0.68 0.68 0.76 0.76 0.84 0.84 0.92 0.92 1]  y_out="[-1 -1  1  1 -1 -1 -1 -1 -1 -1]"
  ri_to_c{1..12} (12 alike) : casper_library_misc/ri_to_c
  sqrt : xbsIndex_r4/Black Box  init_code=sqrt_config  sim_method=ISE Simulator  verbose=off  block_type=blackbox2
  sqrt1 : xbsIndex_r4/Black Box  init_code=sqrt_config  sim_method=ISE Simulator  verbose=off  block_type=blackbox2
  tracex1 : xbsIndex_r4/AddSub  mode=Addition  use_carryin=off  use_carryout=off  en=off  latency=0  precision=Full  arith_type="Signed  (2's comp)"  n_bits=64  bin_pt=26  quantization="Round  (unbiased: +/- Inf)"  overflow=Wrap  dbl_ovrd=off  use_behavioral_HDL=off  hw_selection=Fabric  pipelined=off  block_type=addsub
  tracex10 : xbsIndex_r4/AddSub  mode=Subtraction  use_carryin=off  use_carryout=off  en=off  latency=1  precision=Full  arith_type="Signed  (2's comp)"  n_bits=64  bin_pt=26  quantization="Round  (unbiased: +/- Inf)"  overflow=Wrap  dbl_ovrd=off  use_behavioral_HDL=off  hw_selection=Fabric  pipelined=off  block_type=addsub
  tracex2 : xbsIndex_r4/AddSub  mode=Addition  use_carryin=off  use_carryout=off  en=off  latency=0  precision=Full  arith_type=Unsigned  n_bits=8  bin_pt=0  quantization="Round  (unbiased: +/- Inf)"  overflow=Saturate  dbl_ovrd=off  use_behavioral_HDL=off  hw_selection=Fabric  pipelined=off  block_type=addsub
  tracex3 : xbsIndex_r4/AddSub  mode=Addition  use_carryin=off  use_carryout=off  en=on  latency=1  precision=Full  arith_type="Signed  (2's comp)"  n_bits=64  bin_pt=26  quantization="Round  (unbiased: +/- Inf)"  overflow=Wrap  dbl_ovrd=off  use_behavioral_HDL=off  hw_selection=Fabric  pipelined=off  block_type=addsub
  tracex4 : xbsIndex_r4/AddSub  mode=Subtraction  use_carryin=off  use_carryout=off  en=on  latency=1  precision=Full  arith_type="Signed  (2's comp)"  n_bits=64  bin_pt=26  quantization="Round  (unbiased: +/- Inf)"  overflow=Wrap  dbl_ovrd=off  use_behavioral_HDL=off  hw_selection=Fabric  pipelined=off  block_type=addsub
  tracex5 : xbsIndex_r4/AddSub  mode=Subtraction  use_carryin=off  use_carryout=off  en=off  latency=1  precision=Full  arith_type="Signed  (2's comp)"  n_bits=64  bin_pt=26  quantization="Round  (unbiased: +/- Inf)"  overflow=Wrap  dbl_ovrd=off  use_behavioral_HDL=off  hw_selection=Fabric  pipelined=off  block_type=addsub
  tracex6 : xbsIndex_r4/AddSub  mode=Addition  use_carryin=off  use_carryout=off  en=off  latency=0  precision=Full  arith_type="Signed  (2's comp)"  n_bits=64  bin_pt=26  quantization="Round  (unbiased: +/- Inf)"  overflow=Wrap  dbl_ovrd=off  use_behavioral_HDL=off  hw_selection=Fabric  pipelined=off  block_type=addsub
  tracex7 : xbsIndex_r4/AddSub  mode=Addition  use_carryin=off  use_carryout=off  en=off  latency=0  precision=Full  arith_type=Unsigned  n_bits=8  bin_pt=0  quantization="Round  (unbiased: +/- Inf)"  overflow=Saturate  dbl_ovrd=off  use_behavioral_HDL=off  hw_selection=Fabric  pipelined=off  block_type=addsub
  tracex8 : xbsIndex_r4/AddSub  mode=Addition  use_carryin=off  use_carryout=off  en=on  latency=1  precision=Full  arith_type="Signed  (2's comp)"  n_bits=64  bin_pt=26  quantization="Round  (unbiased: +/- Inf)"  overflow=Wrap  dbl_ovrd=off  use_behavioral_HDL=off  hw_selection=Fabric  pipelined=off  block_type=addsub
  tracex9 : xbsIndex_r4/AddSub  mode=Subtraction  use_carryin=off  use_carryout=off  en=on  latency=1  precision=Full  arith_type="Signed  (2's comp)"  n_bits=64  bin_pt=26  quantization="Round  (unbiased: +/- Inf)"  overflow=Wrap  dbl_ovrd=off  use_behavioral_HDL=off  hw_selection=Fabric  pipelined=off  block_type=addsub
  wires:
  [co_ch0] -> comp_addsub/1(a), comp_addsub1/2(b)
  [co_ch0] -> comp_addsub3/2(b), comp_addsub2/1(a)
  [cy_ch0] -> comp_addsub3/1(a), comp_addsub2/2(b)
  comp_addsub/1(out) -> c_to_ri/1
  c_to_ri/1 -> Reinterpret11/1
  c_to_ri/2 -> Reinterpret12/1
  comp_addsub1/1(out) -> c_to_ri1/1
  comp_addsub2/1(out) -> c_to_ri2/1
  comp_addsub3/1(out) -> c_to_ri3/1
  c_to_ri1/1 -> Reinterpret13/1
  c_to_ri1/2 -> Reinterpret26/1
  c_to_ri2/1 -> Reinterpret27/1
  c_to_ri2/2 -> Reinterpret28/1
  c_to_ri3/1 -> Reinterpret29/1
  c_to_ri3/2 -> Reinterpret30/1
  [Nacc] -> Subsystem4/3(Nacc), Subsystem17/3(Nacc), Subsystem16/3(Nacc)
  [rst] -> Subsystem4/5(rst), Subsystem17/5(rst), Subsystem16/5(rst)
  Mult0/1 -> Convert20/1
  [en] -> Subsystem4/4(en), Subsystem17/4(en), Subsystem16/4(en)
  [x1re_ch0] -> Mult0/2, Mult0/1
  [x1im_ch0] -> Mult1/2, Mult1/1
  [x1re_ch0] -> Mult3/1
  [x2re_ch0] -> Mult3/2
  [x2re_ch0] -> Mult5/2, Mult5/1
  [x1im_ch0] -> Mult2/1
  [x2im_ch0] -> Mult2/2
  [x2im_ch0] -> Mult4/2, Mult4/1
  Subsystem16/1(Outacc) -> Mult14/1
  Subsystem16/2(Outen) -> [accdone], Mx22/2, Mx12/2, Mx11/2
  Constant21/1 -> [Nacc]
  Constant/1 -> edge_detect1/1, [en]
  edge_detect1/1 -> [rst]
  Convert7/1 -> [x2im_ch0]
  Convert18/1 -> [y2im_ch0]
  Reinterpret5/1 -> Convert2/1
  Convert2/1 -> Reinterpret6/1
  Subsystem17/1(Outacc) -> Mult15/1
  Subsystem4/1(Outacc) -> Mult16/1
  Reinterpret6/1 -> Mx11/1
  Reinterpret8/1 -> Mx12/1
  Reinterpret10/1 -> Mx22/1
  Mx11/1 -> tracex1/1, Delay2/1, a_c1/1
  Mx22/1 -> a_c1/2, tracex1/2
  Convert/1 -> Reinterpret2/1
  Mx12/1 -> Delay5/1, Mult12/2, Mult12/1
  Mult13/1 -> tracex2/1
  Mult12/1 -> tracex2/2
  a_c1/1 -> Reinterpret1/1
  sqrt/1 -> Reinterpret/1
  sqrt/2 -> Convert8/1
  Constant2/1 -> sqrt/2
  Reinterpret4/1 -> Delay/1
  tracex3/1 -> Convert26/1
  tracex4/1 -> Convert38/1
  tracex2/1 -> sqrt/1
  Convert8/1 -> tracex3/3, tracex4/3
  Reinterpret/1 -> tracex4/2, tracex3/1
  Reinterpret1/1 -> Convert/1
  Reinterpret2/1 -> Mult13/2, Mult13/1
  Convert1/1 -> Reinterpret4/1
  Reinterpret3/1 -> Convert1/1
  tracex1/1 -> Reinterpret3/1
  Delay/1 -> Delay1/1
  Delay1/1 -> tracex4/1, tracex3/2
  Mult1/1 -> Convert21/1
  Mult3/1 -> Convert11/1
  Mult2/1 -> Convert22/1
  Mult5/1 -> Convert23/1
  Mult4/1 -> Convert72/1
  Reinterpret7/1 -> Convert3/1
  Convert3/1 -> Reinterpret8/1
  Reinterpret9/1 -> Convert4/1
  Convert4/1 -> Reinterpret10/1
  [cx_ch0] -> comp_addsub/2(b), comp_addsub1/1(a)
  Reinterpret11/1 -> Convert5/1
  Convert5/1 -> [x1re_ch0]
  Convert6/1 -> [x1im_ch0]
  Reinterpret12/1 -> Convert6/1
  Reinterpret13/1 -> Convert7/1
  Convert15/1 -> Negate/1
  Reinterpret26/1 -> Convert15/1
  Reinterpret27/1 -> Convert16/1
  Convert16/1 -> [y1re_ch0]
  Reinterpret28/1 -> Convert17/1
  Convert17/1 -> [y1im_ch0]
  Reinterpret29/1 -> Convert18/1
  Convert19/1 -> Negate1/1
  Reinterpret30/1 -> Convert19/1
  Negate/1 -> [x2re_ch0]
  Negate1/1 -> [y2re_ch0]
  [ax] -> tracex5/1
  [lamb1x] -> tracex5/2
  Reinterpret15/1 -> Convert27/1
  Convert26/1 -> Reinterpret15/1
  Convert27/1 -> Reinterpret16/1
  Reinterpret16/1 -> [lamb1x]
  bus_create/1(bus_out) -> arctan/1
  [en] -> arctan/2
  tracex5/1 -> bus_create/1(in1)
  [bx] -> bus_create/2(in2)
  arctan/1 -> Reinterpret17/1
  Constant3/1 -> Relational/1
  Constant4/1 -> Relational1/1
  Relational1/1 -> Logical1/1
  Relational/1 -> Logical1/2
  Convert28/1 -> Reinterpret18/1, Negate2/1
  Logical1/1 -> Black Box/2
  Black Box/1 -> Reinterpret14/1
  Reinterpret17/1 -> Convert28/1, Relational2/1, Relational1/2, Relational/2
  Delay2/1 -> [ax]
  Delay5/1 -> [bx]
  Constant5/1 -> Relational2/2
  Relational2/1 -> Mux1/1, Mux/1
  Mux/1 -> Black Box/1
  Negate2/1 -> Reinterpret19/1
  Reinterpret14/1 -> Negate3/1, Mux1/2
  Negate3/1 -> Mux1/3
  Mux1/1 -> [doax]
  Mult6/1 -> Convert29/1
  Mult7/1 -> Convert30/1
  Mult8/1 -> Convert33/1
  Mult9/1 -> Convert31/1
  Mult10/1 -> Convert34/1
  Mult11/1 -> Convert32/1
  [x11_ch01] -> Mult6/1
  [x11_ch23] -> Mult7/1
  [x12_ch01] -> Mult8/1
  [x12_ch23] -> Mult9/1
  [x22_ch01] -> Mult10/1
  [x22_ch23] -> Mult11/1
  [gain1] -> Mult11/2, Mult10/2, Mult9/2, Mult8/2, Mult7/2, Mult6/2
  Convert29/1 -> Subsystem16/1(re)
  Convert30/1 -> Subsystem16/2(im)
  Convert31/1 -> Subsystem17/2(im)
  Convert32/1 -> Subsystem4/2(im)
  Convert33/1 -> Subsystem17/1(re)
  Convert34/1 -> Subsystem4/1(re)
  Mult14/1 -> Convert35/1
  Mult15/1 -> Convert36/1
  Mult16/1 -> Convert37/1
  [gain2] -> Mult16/2, Mult15/2, Mult14/2
  Constant13/1 -> [gain2], [gain1], [gain0]
  Convert35/1 -> Reinterpret5/1
  Convert36/1 -> Reinterpret7/1
  Convert37/1 -> Reinterpret9/1
  Reinterpret20/1 -> Convert39/1
  Convert38/1 -> Reinterpret20/1
  Convert39/1 -> Reinterpret21/1
  Reinterpret21/1 -> [lamb2x]
  Reinterpret18/1 -> Mux/2
  Reinterpret19/1 -> Mux/3
  [snr] -> Mult/1
  [lamb2x] -> Mult/2
  [lamb1x] -> Delay10/1
  Mult/1 -> Relational3/2
  AddSub/1 -> Register/1
  Register/1 -> AddSub/2, Shift/1
  [doax] -> AddSub/1
  Relational3/1 -> Convert40/1
  AddSub1/1 -> Register1/1
  Register1/1 -> Relational4/2, AddSub1/2
  Constant6/1 -> Relational4/1
  Relational4/1 -> [doaxvalid], Delay9/1, Register1/2, Register/2
  Shift/1 -> [doaxacc]
  [accdone] -> Delay6/1
  Delay6/1 -> Delay7/1
  Delay7/1 -> Delay8/1
  Delay8/1 -> [accdone2]
  [accdone3] -> AddSub/3
  Logical/1 -> AddSub1/3
  [accdone2] -> Delay11/1
  Delay9/1 -> Mux2/1, Logical/2
  Delay10/1 -> Relational3/1
  Delay11/1 -> Logical/1
  Mux2/1 -> AddSub1/1
  Convert40/1 -> Mux2/2
  Constant7/1 -> Mux2/3
  ri_to_c3/1 -> [co_ch0]
  ri_to_c4/1 -> [cx_ch0]
  ri_to_c5/1 -> [cy_ch0]
  ri_to_c1/1 -> [co_ch1]
  ri_to_c2/1 -> [cx_ch1]
  ri_to_c6/1 -> [cy_ch1]
  ri_to_c9/1 -> [co_ch2]
  ri_to_c10/1 -> [cx_ch2]
  ri_to_c11/1 -> [cy_ch2]
  ri_to_c7/1 -> [co_ch3]
  ri_to_c8/1 -> [cx_ch3]
  ri_to_c12/1 -> [cy_ch3]
  Mult17/1 -> Convert70/1
  [x1re_ch1] -> Mult17/1, Mult17/2
  [x1im_ch1] -> Mult18/1, Mult18/2
  [x1re_ch1] -> Mult20/1
  [x2re_ch1] -> Mult20/2
  [x2re_ch1] -> Mult22/1, Mult22/2
  [x1im_ch1] -> Mult19/1
  [x2im_ch1] -> Mult19/2
  [x2im_ch1] -> Mult21/1, Mult21/2
  Mult18/1 -> Convert83/1
  Mult20/1 -> Convert12/1
  Mult19/1 -> Convert24/1
  Mult22/1 -> Convert25/1
  Mult21/1 -> Convert73/1
  Mult23/1 -> Convert71/1
  [x1re_ch2] -> Mult23/1, Mult23/2
  [x1im_ch2] -> Mult24/1, Mult24/2
  [x1re_ch2] -> Mult32/1
  [x2re_ch2] -> Mult32/2
  [x2re_ch2] -> Mult34/1, Mult34/2
  [x1im_ch2] -> Mult28/1
  [x2im_ch2] -> Mult28/2
  [x2im_ch2] -> Mult33/1, Mult33/2
  Mult24/1 -> Convert93/1
  Mult32/1 -> Convert13/1
  Mult28/1 -> Convert66/1
  Mult34/1 -> Convert68/1
  Mult33/1 -> Convert74/1
  Mult25/1 -> Convert82/1
  [x1re_ch3] -> Mult25/2, Mult25/1
  [x1im_ch3] -> Mult26/2, Mult26/1
  [x1re_ch3] -> Mult29/1
  [x2re_ch3] -> Mult29/2
  [x2re_ch3] -> Mult31/2, Mult31/1
  [x1im_ch3] -> Mult27/1
  [x2im_ch3] -> Mult27/2
  [x2im_ch3] -> Mult30/2, Mult30/1
  Mult26/1 -> Convert94/1
  Mult29/1 -> Convert14/1
  Mult27/1 -> Convert67/1
  Mult31/1 -> Convert69/1
  Mult30/1 -> Convert75/1
  Convert20/1 -> AddSub2/1
  Convert21/1 -> AddSub2/2
  Convert70/1 -> AddSub3/1
  Convert83/1 -> AddSub3/2
  Convert71/1 -> AddSub4/1
  Convert93/1 -> AddSub4/2
  Convert82/1 -> AddSub5/1
  Convert94/1 -> AddSub5/2
  AddSub2/1 -> AddSub6/1
  AddSub3/1 -> AddSub6/2
  AddSub4/1 -> AddSub7/1
  AddSub5/1 -> AddSub7/2
  AddSub8/1 -> AddSub12/1
  AddSub9/1 -> AddSub12/2
  AddSub10/1 -> AddSub13/1
  AddSub11/1 -> AddSub13/2
  Convert11/1 -> AddSub8/1
  Convert22/1 -> AddSub8/2
  Convert12/1 -> AddSub9/1
  Convert24/1 -> AddSub9/2
  Convert13/1 -> AddSub10/1
  Convert66/1 -> AddSub10/2
  Convert14/1 -> AddSub11/1
  Convert67/1 -> AddSub11/2
  AddSub18/1 -> AddSub16/1
  AddSub19/1 -> AddSub16/2
  AddSub14/1 -> AddSub17/1
  AddSub15/1 -> AddSub17/2
  Convert23/1 -> AddSub18/1
  Convert72/1 -> AddSub18/2
  Convert25/1 -> AddSub19/1
  Convert73/1 -> AddSub19/2
  Convert68/1 -> AddSub14/1
  Convert74/1 -> AddSub14/2
  Convert69/1 -> AddSub15/1
  Convert75/1 -> AddSub15/2
  AddSub6/1 -> [x11_ch01]
  AddSub7/1 -> [x11_ch23]
  AddSub12/1 -> [x12_ch01]
  AddSub13/1 -> [x12_ch23]
  AddSub16/1 -> [x22_ch01]
  AddSub17/1 -> [x22_ch23]
  [gain0] -> Mult46/1, Mult45/1, Mult44/1, Mult43/1, Mult42/1, Mult41/1, Mult40/1, Mult39/1, Mult38/1, Mult37/1, Mult36/1, Mult35/1
  [ch0re_a1] -> Mult35/2
  [ch0im_a1] -> Mult36/2
  Mult35/1 -> Convert9/1
  Mult36/1 -> Convert10/1
  Convert10/1 -> ri_to_c3/2
  Convert9/1 -> ri_to_c3/1
  [ch0re_a2] -> Mult37/2
  [ch0im_a2] -> Mult38/2
  [ch0re_a3] -> Mult39/2
  [ch0im_a3] -> Mult40/2
  [ch1re_a1] -> Mult41/2
  [ch1im_a1] -> Mult42/2
  [ch1re_a2] -> Mult43/2
  [ch1im_a2] -> Mult44/2
  [ch1re_a3] -> Mult45/2
  [ch1im_a3] -> Mult46/2
  Mult37/1 -> Convert76/1
  Convert76/1 -> ri_to_c4/1
  Mult38/1 -> Convert65/1
  Convert65/1 -> ri_to_c4/2
  Mult39/1 -> Convert88/1
  Convert88/1 -> ri_to_c5/1
  Mult40/1 -> Convert77/1
  Convert77/1 -> ri_to_c5/2
  Mult41/1 -> Convert100/1
  Convert100/1 -> ri_to_c1/1
  Mult42/1 -> Convert99/1
  Convert99/1 -> ri_to_c1/2
  Mult43/1 -> Convert101/1
  Convert101/1 -> ri_to_c2/1
  Mult44/1 -> Convert102/1
  Convert102/1 -> ri_to_c2/2
  Convert103/1 -> ri_to_c6/1
  Mult45/1 -> Convert103/1
  Mult46/1 -> Convert104/1
  Convert104/1 -> ri_to_c6/2
  [gain0] -> Mult47/1, Mult48/1, Mult49/1, Mult50/1, Mult51/1, Mult52/1, Mult53/1, Mult54/1, Mult55/1, Mult56/1, Mult57/1, Mult58/1
  [ch2re_a1] -> Mult47/2
  [ch2im_a1] -> Mult48/2
  Mult47/1 -> Convert115/1
  Mult48/1 -> Convert105/1
  Convert105/1 -> ri_to_c9/2
  Convert115/1 -> ri_to_c9/1
  [ch2re_a2] -> Mult49/2
  [ch2im_a2] -> Mult50/2
  [ch2re_a3] -> Mult51/2
  [ch2im_a3] -> Mult52/2
  [ch3re_a1] -> Mult53/2
  [ch3im_a1] -> Mult54/2
  [ch3re_a2] -> Mult55/2
  [ch3im_a2] -> Mult56/2
  [ch3re_a3] -> Mult57/2
  [ch3im_a3] -> Mult58/2
  Mult49/1 -> Convert112/1
  Convert112/1 -> ri_to_c10/1
  Mult50/1 -> Convert111/1
  Convert111/1 -> ri_to_c10/2
  Mult51/1 -> Convert114/1
  Convert114/1 -> ri_to_c11/1
  Mult52/1 -> Convert113/1
  Convert113/1 -> ri_to_c11/2
  Mult53/1 -> Convert106/1
  Convert106/1 -> ri_to_c7/1
  Mult54/1 -> Convert116/1
  Convert116/1 -> ri_to_c7/2
  Mult55/1 -> Convert107/1
  Convert107/1 -> ri_to_c8/1
  Mult56/1 -> Convert108/1
  Convert108/1 -> ri_to_c8/2
  Convert109/1 -> ri_to_c12/1
  Mult57/1 -> Convert109/1
  Mult58/1 -> Convert110/1
  Convert110/1 -> ri_to_c12/2
  [co_ch2] -> comp_addsub9/2(b), comp_addsub8/1(a)
  [co_ch2] -> comp_addsub10/1(a), comp_addsub11/2(b)
  [cy_ch2] -> comp_addsub10/2(b), comp_addsub11/1(a)
  comp_addsub8/1(out) -> c_to_ri8/1
  c_to_ri8/1 -> Reinterpret35/1
  c_to_ri8/2 -> Reinterpret36/1
  comp_addsub9/1(out) -> c_to_ri9/1
  comp_addsub10/1(out) -> c_to_ri10/1
  comp_addsub11/1(out) -> c_to_ri11/1
  c_to_ri9/1 -> Reinterpret37/1
  c_to_ri9/2 -> Reinterpret42/1
  c_to_ri10/1 -> Reinterpret43/1
  c_to_ri10/2 -> Reinterpret44/1
  c_to_ri11/1 -> Reinterpret45/1
  c_to_ri11/2 -> Reinterpret46/1
  Convert64/1 -> [x2im_ch2]
  Convert52/1 -> [y2im_ch2]
  [cx_ch2] -> comp_addsub9/1(a), comp_addsub8/2(b)
  Reinterpret35/1 -> Convert62/1
  Convert62/1 -> [x1re_ch2]
  Convert63/1 -> [x1im_ch2]
  Reinterpret36/1 -> Convert63/1
  Reinterpret37/1 -> Convert64/1
  Convert49/1 -> Negate6/1
  Reinterpret42/1 -> Convert49/1
  Reinterpret43/1 -> Convert50/1
  Convert50/1 -> [y1re_ch2]
  Reinterpret44/1 -> Convert51/1
  Convert51/1 -> [y1im_ch2]
  Reinterpret45/1 -> Convert52/1
  Convert53/1 -> Negate7/1
  Reinterpret46/1 -> Convert53/1
  Negate6/1 -> [x2re_ch2]
  Negate7/1 -> [y2re_ch2]
  [co_ch1] -> comp_addsub5/2(b), comp_addsub4/1(a)
  [co_ch1] -> comp_addsub6/1(a), comp_addsub7/2(b)
  [cy_ch1] -> comp_addsub6/2(b), comp_addsub7/1(a)
  comp_addsub4/1(out) -> c_to_ri4/1
  c_to_ri4/1 -> Reinterpret22/1
  c_to_ri4/2 -> Reinterpret23/1
  comp_addsub5/1(out) -> c_to_ri5/1
  comp_addsub6/1(out) -> c_to_ri6/1
  comp_addsub7/1(out) -> c_to_ri7/1
  c_to_ri5/1 -> Reinterpret24/1
  c_to_ri5/2 -> Reinterpret25/1
  c_to_ri6/1 -> Reinterpret31/1
  c_to_ri6/2 -> Reinterpret32/1
  c_to_ri7/1 -> Reinterpret33/1
  c_to_ri7/2 -> Reinterpret34/1
  Convert48/1 -> [x2im_ch1]
  Convert44/1 -> [y2im_ch1]
  [cx_ch1] -> comp_addsub5/1(a), comp_addsub4/2(b)
  Reinterpret22/1 -> Convert46/1
  Convert46/1 -> [x1re_ch1]
  Convert47/1 -> [x1im_ch1]
  Reinterpret23/1 -> Convert47/1
  Reinterpret24/1 -> Convert48/1
  Convert41/1 -> Negate4/1
  Reinterpret25/1 -> Convert41/1
  Reinterpret31/1 -> Convert42/1
  Convert42/1 -> [y1re_ch1]
  Reinterpret32/1 -> Convert43/1
  Convert43/1 -> [y1im_ch1]
  Reinterpret33/1 -> Convert44/1
  Convert45/1 -> Negate5/1
  Reinterpret34/1 -> Convert45/1
  Negate4/1 -> [x2re_ch1]
  Negate5/1 -> [y2re_ch1]
  [co_ch3] -> comp_addsub12/1(a), comp_addsub13/2(b)
  [co_ch3] -> comp_addsub15/2(b), comp_addsub14/1(a)
  [cy_ch3] -> comp_addsub15/1(a), comp_addsub14/2(b)
  comp_addsub12/1(out) -> c_to_ri12/1
  c_to_ri12/1 -> Reinterpret38/1
  c_to_ri12/2 -> Reinterpret39/1
  comp_addsub13/1(out) -> c_to_ri13/1
  comp_addsub14/1(out) -> c_to_ri14/1
  comp_addsub15/1(out) -> c_to_ri15/1
  c_to_ri13/1 -> Reinterpret40/1
  c_to_ri13/2 -> Reinterpret41/1
  c_to_ri14/1 -> Reinterpret47/1
  c_to_ri14/2 -> Reinterpret48/1
  c_to_ri15/1 -> Reinterpret49/1
  c_to_ri15/2 -> Reinterpret50/1
  Convert61/1 -> [x2im_ch3]
  Convert57/1 -> [y2im_ch3]
  [cx_ch3] -> comp_addsub12/2(b), comp_addsub13/1(a)
  Reinterpret38/1 -> Convert59/1
  Convert59/1 -> [x1re_ch3]
  Convert60/1 -> [x1im_ch3]
  Reinterpret39/1 -> Convert60/1
  Reinterpret40/1 -> Convert61/1
  Convert54/1 -> Negate8/1
  Reinterpret41/1 -> Convert54/1
  Reinterpret47/1 -> Convert55/1
  Convert55/1 -> [y1re_ch3]
  Reinterpret48/1 -> Convert56/1
  Convert56/1 -> [y1im_ch3]
  Reinterpret49/1 -> Convert57/1
  Convert58/1 -> Negate9/1
  Reinterpret50/1 -> Convert58/1
  Negate8/1 -> [x2re_ch3]
  Negate9/1 -> [y2re_ch3]
  Mult59/1 -> Convert84/1
  [y1re_ch0] -> Mult59/1, Mult59/2
  [y1im_ch0] -> Mult60/1, Mult60/2
  [y1re_ch0] -> Mult75/1
  [y2re_ch0] -> Mult75/2
  [y2re_ch0] -> Mult82/1, Mult82/2
  [y1im_ch0] -> Mult64/1
  [y2im_ch0] -> Mult64/2
  [y2im_ch0] -> Mult81/1, Mult81/2
  Mult60/1 -> Convert85/1
  Mult75/1 -> Convert78/1
  Mult64/1 -> Convert86/1
  Mult82/1 -> Convert87/1
  Mult81/1 -> Convert117/1
  Mult61/1 -> Convert97/1
  [y1re_ch1] -> Mult61/2, Mult61/1
  [y1im_ch1] -> Mult62/2, Mult62/1
  [y1re_ch1] -> Mult65/1
  [y2re_ch1] -> Mult65/2
  [y2re_ch1] -> Mult67/2, Mult67/1
  [y1im_ch1] -> Mult63/1
  [y2im_ch1] -> Mult63/2
  [y2im_ch1] -> Mult66/2, Mult66/1
  Mult62/1 -> Convert122/1
  Mult65/1 -> Convert79/1
  Mult63/1 -> Convert89/1
  Mult67/1 -> Convert90/1
  Mult66/1 -> Convert118/1
  Mult68/1 -> Convert98/1
  [y1re_ch2] -> Mult68/2, Mult68/1
  [y1im_ch2] -> Mult69/2, Mult69/1
  [y1re_ch2] -> Mult78/1
  [y2re_ch2] -> Mult78/2
  [y2re_ch2] -> Mult80/2, Mult80/1
  [y1im_ch2] -> Mult73/1
  [y2im_ch2] -> Mult73/2
  [y2im_ch2] -> Mult79/2, Mult79/1
  Mult69/1 -> Convert123/1
  Mult78/1 -> Convert80/1
  Mult73/1 -> Convert91/1
  Mult80/1 -> Convert95/1
  Mult79/1 -> Convert119/1
  Mult70/1 -> Convert121/1
  [y1re_ch3] -> Mult70/1, Mult70/2
  [y1im_ch3] -> Mult71/1, Mult71/2
  [y1re_ch3] -> Mult74/1
  [y2re_ch3] -> Mult74/2
  [y2re_ch3] -> Mult77/1, Mult77/2
  [y1im_ch3] -> Mult72/1
  [y2im_ch3] -> Mult72/2
  [y2im_ch3] -> Mult76/1, Mult76/2
  Mult71/1 -> Convert124/1
  Mult74/1 -> Convert81/1
  Mult72/1 -> Convert92/1
  Mult77/1 -> Convert96/1
  Mult76/1 -> Convert120/1
  Convert84/1 -> AddSub30/1
  Convert85/1 -> AddSub30/2
  Convert97/1 -> AddSub31/1
  Convert122/1 -> AddSub31/2
  Convert98/1 -> AddSub32/1
  Convert123/1 -> AddSub32/2
  Convert121/1 -> AddSub33/1
  Convert124/1 -> AddSub33/2
  AddSub30/1 -> AddSub34/1
  AddSub31/1 -> AddSub34/2
  AddSub32/1 -> AddSub35/1
  AddSub33/1 -> AddSub35/2
  AddSub36/1 -> AddSub22/1
  AddSub37/1 -> AddSub22/2
  AddSub20/1 -> AddSub23/1
  AddSub21/1 -> AddSub23/2
  Convert78/1 -> AddSub36/1
  Convert86/1 -> AddSub36/2
  Convert79/1 -> AddSub37/1
  Convert89/1 -> AddSub37/2
  Convert80/1 -> AddSub20/1
  Convert91/1 -> AddSub20/2
  Convert81/1 -> AddSub21/1
  Convert92/1 -> AddSub21/2
  AddSub28/1 -> AddSub26/1
  AddSub29/1 -> AddSub26/2
  AddSub24/1 -> AddSub27/1
  AddSub25/1 -> AddSub27/2
  Convert87/1 -> AddSub28/1
  Convert117/1 -> AddSub28/2
  Convert90/1 -> AddSub29/1
  Convert118/1 -> AddSub29/2
  Convert95/1 -> AddSub24/1
  Convert119/1 -> AddSub24/2
  Convert96/1 -> AddSub25/1
  Convert120/1 -> AddSub25/2
  AddSub34/1 -> [y11_ch01]
  AddSub35/1 -> [y11_ch23]
  AddSub22/1 -> [y12_ch01]
  AddSub23/1 -> [y12_ch23]
  AddSub26/1 -> [y22_ch01]
  AddSub27/1 -> [y22_ch23]
  arctan/2 -> Terminator/1
  [Nacc] -> Subsystem1/3(Nacc), Subsystem2/3(Nacc), Subsystem3/3(Nacc)
  [rst] -> Subsystem1/5(rst), Subsystem2/5(rst), Subsystem3/5(rst)
  [en] -> Subsystem1/4(en), Subsystem2/4(en), Subsystem3/4(en)
  Subsystem1/1(Outacc) -> Mult87/1
  Subsystem1/2(Outen) -> Mx1/2, Mx2/2, Mx3/2
  Reinterpret61/1 -> Convert127/1
  Convert127/1 -> Reinterpret62/1
  Subsystem2/1(Outacc) -> Mult88/1
  Subsystem3/1(Outacc) -> Mult89/1
  Reinterpret62/1 -> Mx1/1
  Reinterpret64/1 -> Mx2/1
  Reinterpret53/1 -> Mx3/1
  Mx1/1 -> a_c2/1, Delay12/1, tracex6/1
  Mx3/1 -> tracex6/2, a_c2/2
  Convert125/1 -> Reinterpret56/1
  Mx2/1 -> Mult85/1, Mult85/2, Delay13/1
  Mult86/1 -> tracex7/1
  Mult85/1 -> tracex7/2
  a_c2/1 -> Reinterpret52/1
  sqrt1/1 -> Reinterpret51/1
  sqrt1/2 -> Convert143/1
  Constant1/1 -> sqrt1/2
  Reinterpret60/1 -> Delay3/1
  tracex8/1 -> Convert128/1
  tracex9/1 -> Convert140/1
  tracex7/1 -> sqrt1/1
  Convert143/1 -> tracex9/3, tracex8/3
  Reinterpret51/1 -> tracex8/1, tracex9/2
  Reinterpret52/1 -> Convert125/1
  Reinterpret56/1 -> Mult86/1, Mult86/2
  Convert126/1 -> Reinterpret60/1
  Reinterpret59/1 -> Convert126/1
  tracex6/1 -> Reinterpret59/1
  Delay3/1 -> Delay4/1
  Delay4/1 -> tracex8/2, tracex9/1
  Reinterpret63/1 -> Convert131/1
  Convert131/1 -> Reinterpret64/1
  Reinterpret65/1 -> Convert142/1
  Convert142/1 -> Reinterpret53/1
  Reinterpret54/1 -> Convert129/1
  Convert128/1 -> Reinterpret54/1
  Convert129/1 -> Reinterpret55/1
  Reinterpret55/1 -> [lamb1y]
  Delay12/1 -> [ay]
  Delay13/1 -> [by]
  Mult90/1 -> Convert130/1
  Mult91/1 -> Convert132/1
  Mult92/1 -> Convert135/1
  Mult93/1 -> Convert133/1
  Mult83/1 -> Convert136/1
  Mult84/1 -> Convert134/1
  [y11_ch01] -> Mult90/1
  [y11_ch23] -> Mult91/1
  [y12_ch01] -> Mult92/1
  [y12_ch23] -> Mult93/1
  [y22_ch01] -> Mult83/1
  [y22_ch23] -> Mult84/1
  [gain1] -> Mult90/2, Mult91/2, Mult92/2, Mult93/2, Mult83/2, Mult84/2
  Convert130/1 -> Subsystem1/1(re)
  Convert132/1 -> Subsystem1/2(im)
  Convert133/1 -> Subsystem2/2(im)
  Convert134/1 -> Subsystem3/2(im)
  Convert135/1 -> Subsystem2/1(re)
  Convert136/1 -> Subsystem3/1(re)
  Mult87/1 -> Convert137/1
  Mult88/1 -> Convert138/1
  Mult89/1 -> Convert139/1
  [gain2] -> Mult87/2, Mult88/2, Mult89/2
  Convert137/1 -> Reinterpret61/1
  Convert138/1 -> Reinterpret63/1
  Convert139/1 -> Reinterpret65/1
  Reinterpret57/1 -> Convert141/1
  Convert140/1 -> Reinterpret57/1
  Convert141/1 -> Reinterpret58/1
  Reinterpret58/1 -> [lamb2y]
  [ay] -> tracex10/1
  [lamb1y] -> tracex10/2
  bus_create1/1(bus_out) -> arctan1/1
  [en] -> arctan1/2
  tracex10/1 -> bus_create1/1(in1)
  [by] -> bus_create1/2(in2)
  arctan1/1 -> Reinterpret67/1
  Constant8/1 -> Relational5/1
  Constant9/1 -> Relational6/1
  Relational6/1 -> Logical2/1
  Relational5/1 -> Logical2/2
  Convert144/1 -> Negate10/1, Reinterpret68/1
  Logical2/1 -> Black Box1/2
  Black Box1/1 -> Reinterpret66/1
  Reinterpret67/1 -> Relational5/2, Relational6/2, Relational7/1, Convert144/1
  Constant10/1 -> Relational7/2
  Relational7/1 -> Mux3/1, Mux4/1
  Mux3/1 -> Black Box1/1
  Negate10/1 -> Reinterpret69/1
  Reinterpret66/1 -> Mux4/2, Negate11/1
  Negate11/1 -> Mux4/3
  Mux4/1 -> [doay]
  Reinterpret68/1 -> Mux3/2
  Reinterpret69/1 -> Mux3/3
  arctan1/2 -> Terminator1/1
  [snr] -> Mult94/1
  [lamb2y] -> Mult94/2
  [lamb1y] -> Delay17/1
  Mult94/1 -> Relational8/2
  AddSub38/1 -> Register2/1
  Register2/1 -> Shift1/1, AddSub38/2
  [doay] -> AddSub38/1
  Relational8/1 -> Convert145/1
  AddSub39/1 -> Register3/1
  Register3/1 -> AddSub39/2, Relational9/2
  Constant11/1 -> Relational9/1
  Relational9/1 -> Register2/2, Register3/2, Delay19/1, [doayvalid]
  Shift1/1 -> [doayacc]
  [accdone3] -> AddSub38/3
  Logical3/1 -> AddSub39/3, [accdone3]
  [accdone2] -> Delay18/1
  Delay19/1 -> Logical3/2, Mux5/1
  Delay17/1 -> Relational8/1
  Delay18/1 -> Logical3/1
  Mux5/1 -> AddSub39/1
  Convert145/1 -> Mux5/2
  Constant12/1 -> Mux5/3
  Constant14/1 -> [snr]
  Constant15/1 -> [ch0re_a1], [ch0im_a1], [ch0re_a2], [ch0im_a2], [ch0re_a3], [ch0im_a3], [ch1re_a1], [ch1im_a1], [ch1re_a2], [ch1im_a2], [ch1re_a3], [ch1im_a3], [ch2re_a1], [ch2im_a1], [ch2re_a2], [ch2im_a2], [ch2re_a3], [ch2im_a3], [ch3re_a1], [ch3im_a1], [ch3im_a2], [ch3re_a3], [ch3im_a3], [ch3re_a2]
